simulink model "Question1"  (R2018a)
settings: Solver=VariableStepDiscrete  StartTime=0.0  StopTime=0.4  RelTol=1e-3
libraries: powerlib x9
settings Model: Creator=enes_  LastModifiedBy=bulbu

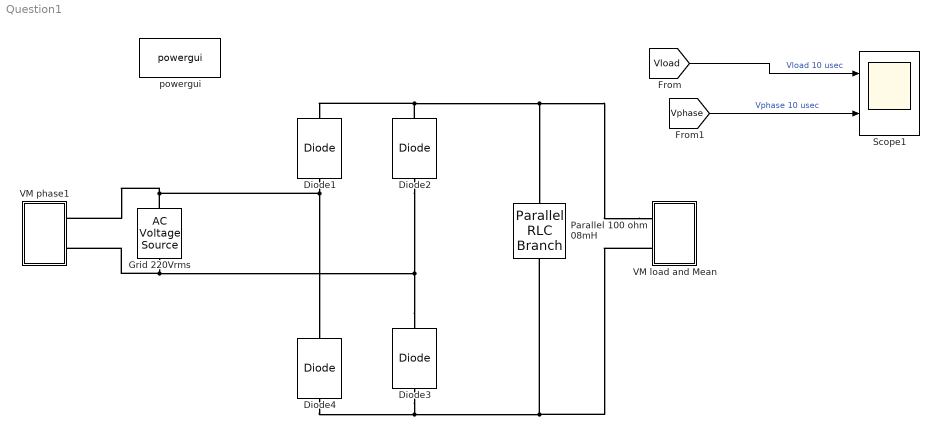
== system Question1 ==
  Diode{1..4} (4 alike) : powerlib/Power Electronics/Diode  Ron=0.001  Lon=0  Vf=0.8  IC=0  UseSnubber=0  Rs=500  Cs=250e-9  Measurements=off
  Grid 220Vrms : powerlib/Electrical Sources/AC Voltage Source  Amplitude=326.6  Phase=0  Frequency=50  SampleTime=0  Measurements=None  BusType=swing  Pref=10e3  Qref=0  Qmin=-inf  Qmax=+inf
  Parallel 100 ohm 08mH : powerlib/Elements/Parallel RLC Branch  LConnTagsString=a  RConnTagsString=__new0  BranchType=R  Resistance=100  Inductance=1e-3  SetiL0=off  InitialCurrent=0  Capacitance=0.8e-3  Setx0=off  InitialVoltage=0  Measurements=None
  Scope1 : Scope  NumInputPorts=2
  VM load and Mean : Subsystem
  VM phase1 : Subsystem
  powergui : powerlib/powergui  Priority=1  SimulationMode=Discrete  SampleTime=10e-6  frequency=60  Iterations=50  frequencyindice=50  Pbase=100e6  ErrMax=1e-4  UnitsV=kV  UnitsW=MW  buscounter=0  FunctionMessages=off  echomessages=off  EnableUseOfTLC=off  CurrentSourceSwitches=off  DisableSnubberDevices=off  DisableRonSwitches=off  DisableVfSwitches=off  DisplayEquations=off  SolverType=Tustin/Backward Euler (TBE)  Interpol=off  ExternalGateDelay=off  methode=off  Ts=100  x0status=blocks  SPID=on  SwTol=0  HookPort=off  RestoreLinks=warning  ResistiveCurrentMeasurement=off  Frange=[0:2:500]  Ylog=off  Xlog=on  ShowGrid=off  save=off  variable=ZData  structure=0  ZoomFFT=off  StartTime=0.0  cycles=1  DisplayStyle=1  fundamental=60  FreqAxis=off  MaxFrequency=1000  frequencyindicesteady=1  RmsSteady=1  display=off
  wires:
  [Vphase] -> Scope1/2  "Vphase 10 usec"
  [Vload] -> Scope1/1  "Vload 10 usec"
  connections:
  Diode3/RConn1 -- Diode2/LConn1 -- Grid 220Vrms/LConn1 -- VM phase1/LConn2
  VM load and Mean/LConn1 -- Parallel 100 ohm 08mH/LConn1 -- Diode2/RConn1 -- Diode1/RConn1
  Parallel 100 ohm 08mH/RConn1 -- VM load and Mean/LConn2 -- Diode3/LConn1 -- Diode4/LConn1
  Diode1/LConn1 -- VM phase1/LConn1 -- Grid 220Vrms/RConn1 -- Diode4/RConn1

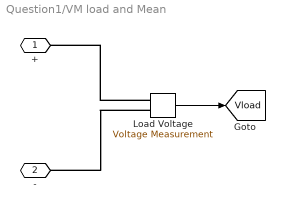
== system Question1/VM load and Mean ==
  Load Voltage : powerlib/Measurements/Voltage Measurement  PhasorSimulation=off  OutputType=Complex  PSBequivalent=0
  + : PMIOPort  Side=Left
  - : PMIOPort  Port=2  Side=Left
  tag scope: Vload=global
  wires:
  Load Voltage/1 -> [Vload]
  connections:
  Load Voltage/LConn1 -- +/RConn1
  Load Voltage/LConn2 -- -/RConn1

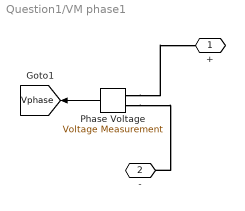
== system Question1/VM phase1 ==
  Phase Voltage : powerlib/Measurements/Voltage Measurement  PhasorSimulation=off  OutputType=Complex  PSBequivalent=0
  + : PMIOPort  Side=Left
  - : PMIOPort  Port=2  Side=Left
  tag scope: Vphase=global
  wires:
  Phase Voltage/1 -> [Vphase]
  connections:
  Phase Voltage/LConn1 -- +/RConn1
  Phase Voltage/LConn2 -- -/RConn1
